simulink model "Phase1_Mark2"  (R2024b)
settings: Solver=ode23tb  StartTime=0.0  StopTime=inf  FixedStep=.001  RelTol=1e-1
model workspace (MAT data in the model file):
  A_mu = 10
  B_reff = 8.386
  CONVERTER_DATA = [0 0.1 0.2 0.3 0.4 0.5 0.6 0.7 0.8 0.81 0.82 0.83 ... (63 elements, 21x3)]
  Cps = 2
  Cz = 7766.25
  DOWN_TABLE = [0 0 0 0 0 0 5 5 7.5 7.5 15 15 ... (30 elements, 6x5)]
  DOWN_TH_BP = [0 5 40 50 90 100]
  D_reff = 0.25826
  EMAP = [-40 215 245 264 264 267 267 267 267 267 -44 117 ... (110 elements, 10x11)]
  F0z = [6086.4 4324.8]
  F_reff = 0.07394
  F_zmax = 10000
  F_zmin = 100
  F_zo = 4000
  Kz = 48000
  MF : object (value not decoded)
  NCyl = 6
  NE_VEC = [800 1200 1600 2000 2400 2800 3200 3600 4000 4400 4800]
  Pstd = 101325
  Rair = 287
  SUS : object (value not decoded)
  TH_VEC = [0; 20; 30; 40; 50; 60; 70; 80; 90; 100]
  TWAITdn = 1.25
  TWAITup = 0.1
  Tin = [1 2 3 4 5 6 7 8 9 10 2 2 ... (20 elements, 10x2)]
  Tstd = 293.15
  UP_TABLE = [7.5 7.5 15 25 40 40 25 25 35 45 70 80 ... (30 elements, 6x5)]
  UP_TH_BP = [0 25 35 50 90 100]
  VEH : object (value not decoded)
  V_o = 16.7
  V_xlow = 1
  Vd = 0.00346
  WH : object (value not decoded)
  a = 1.515
  alpha_max = 1.5
  alpha_min = -1.5
  b = 1.504
  c_zo = 209651
  epsilon = 0.1
  f_air = [0 0 0 0 0 0 0 0 0 0 0 0 ... (256 elements, 16x16)]
  f_co = [0 0 0 0 0 0 0 0 0 0 0 0 ... (256 elements, 16x16)]
  f_co2 = [0 0 0 0 0 0 0 0 0 0 0 0 ... (256 elements, 16x16)]
  f_eff = [352.135682859 352.135682859 320.724378192 303.655312657 295.930136708 291.240087194 291.240271258 291.240312459 291.240275452 291.240198499 291.240100781 291.240018769 ... (256 elements, 16x16)]
  f_fuel = [0 0 0 0 0 0 0 0 0 0 0 0 ... (256 elements, 16x16)]
  f_hc = [0 0 0 0 0 0 0 0 0 0 0 0 ... (256 elements, 16x16)]
  f_nox = [0 0 0 0 0 0 0 0 0 0 0 0 ... (256 elements, 16x16)]
  f_pm = [0 0 0 0 0 0 0 0 0 0 0 0 ... (256 elements, 16x16)]
  f_susp_axl_bp = [1 2]
  f_susp_dz_bp = [-4 -0.14 -0.13 -0.12 -0.11 -0.1 -0.09 -0.08 -0.07 -0.06 -0.05 -0.04 ... (31 elements, 1x31)]
  f_susp_dzdot_bp = [-4 -0.14 -0.13 -0.12 -0.11 -0.1 -0.09 -0.08 -0.07 -0.06 -0.05 -0.04 ... (31 elements, 1x31)]
  f_susp_fmz = [-213379.591456 -28099.591456 -27619.591456 -27139.591456 -26659.591456 -26179.591456 -25699.591456 -25219.591456 -24739.591456 -24259.591456 -23779.591456 -23299.591456 ... (468968 elements, 31x31x61x2x4)]
  f_susp_geom = [-0.832564012244 0.043269987756 0.045538987756 0.047807987756 0.050076987756 0.052345987756 0.054614987756 0.056883987756 0.059152987756 0.061421987756 0.063690987756 0.065959987756 ... (11346 elements, 31x61x2x3)]
  f_susp_strgdelta_bp = [-0.523598775598 -0.506145483078 -0.488692190558 -0.471238898038 -0.453785605519 -0.436332312999 -0.418879020479 -0.401425727959 -0.383972435439 -0.366519142919 -0.349065850399 -0.331612557879 ... (61 elements, 1x61)]
  f_tbrake = [0 76.8593923996 105.140482948 131.533638111 157.926793274 176.658631717 176.65727296 176.656856686 176.656879077 176.657093756 176.657404516 176.65772406 ... (256 elements, 16x16)]
  f_tbrake_n_bpt = [0 649.519052838 912.419621844 1175.32019085 1438.22075986 1701.12132886 1964.02189787 2226.92246687 2489.82303588 2752.72360489 3015.62417389 3278.5247429 ... (16 elements, 1x16)]
  f_tbrake_t_bpt = [0 34.6410161514 61.0341713143 87.4273264773 113.82048164 140.213636803 166.606791966 192.999947129 219.393102292 245.786257455 272.179412618 298.572567781 ... (16 elements, 1x16)]
  f_texh = [766.752464599 766.752464599 786.17542386 801.679939032 884.591982581 910.574397722 910.571871054 910.570774534 910.570601632 910.570821151 910.571247242 910.571639815 ... (256 elements, 16x16)]
  f_twc_eff_co = [0.17 0.25 0.45 0.99 0.99 0.99 0.99]
  f_twc_eff_hc = [0.21 0.375 0.75 0.98 0.98 0.98 0.98]
  f_twc_eff_lam = [0.909090909 0.944055944 0.979020979 1 1.013986014 1.048951049 1.083916084]
  f_twc_eff_nox = [0.98 0.98 0.98 0.97 0.05 0.02 0]
  h = 0.134
  k_z = 50
  kappa_max = 1.5
  kappa_min = -1.5
  lam_Cx = 1
  lam_Cy = 1
  lam_Cz = 1
  lam_Ex = 1
  lam_Ey = 1
  lam_F_zo = 1
  lam_Hx = 1
  lam_Hy = 1
  lam_Kxkappa = 1
  lam_Kyalpha = 1
  lam_Kygamma = 1
  lam_Kzgamma = 1
  lam_Mr = 1
  lam_Mx = 1
  lam_My = 1
  lam_S = 1
  lam_VMx = 1
  lam_Vx = 1
  lam_Vy = 1
  lam_Vykappa = 1
  lam_muV = 0
  lam_mux = 1
  lam_muy = 1
  lam_t = 1
  lam_xalpha = 1
  lam_ykappa = 1
  numWheel = 4
  p_Cx1 = 1.579
  p_Cy1 = 1.3332
  p_Dx1 = 1.0422
  p_Dx2 = -0.08285
  p_Dx3 = 0
  p_Dy1 = 0.8784
  p_Dy2 = -0.06445
  p_Dy3 = 0
  p_Ex1 = 0.11185
  p_Ex2 = 0.3127
  p_Ex3 = 0
  p_Ex4 = 0.001603
  p_Ey1 = -0.8227
  p_Ey2 = -0.6062
  p_Ey3 = 0.09825
  p_Ey4 = -6.546
  p_Ey5 = 0
  p_Fz1 = 0.7098
  p_Hx1 = 0.00021585
  p_Hx2 = 0.0011538
  p_Hy1 = -0.0018043
  p_Hy2 = 0.003518
  p_Kx1 = 21.69
  p_Kx2 = 13.774
  p_Kx3 = -0.4119
  p_Ky1 = -15.314
  p_Ky2 = 1.7044
  p_Ky3 = 0.36986
  p_Ky4 = 1.9896
  p_Ky5 = 0
  p_Ky6 = -0.9004
  p_Ky7 = -0.2328
  p_Vx1 = 1.5973e-05
  p_Vx2 = 0.0001043
  p_Vy1 = -0.006642
  p_Vy2 = 0.03597
  p_Vy3 = -0.1621
  p_Vy4 = -0.4908
  p_pmx1 = 0
  p_px1 = -0.3489
  p_px2 = 0.382
  p_px3 = -0.09634
  p_px4 = 0.06447
  p_py1 = -0.6249
  p_py2 = -0.06535
  p_py3 = -0.1668
  p_py4 = 0.2834
  p_py5 = 0
  path : object (value not decoded)
  pio = 220000
  q_Fcx = 0
  q_Fz2 = 15.4
  q_Fzy = 0
  q_reo = 0.9974
  q_sx1 = -0.007764
  q_sx10 = 0.2824
  q_sx11 = 5.349
  q_sx12 = 0
  q_sx13 = 0
  q_sx14 = 0
  q_sx2 = 1.1915
  q_sx3 = 0.013948
  q_sx4 = 4.912
  q_sx5 = 1.02
  q_sx6 = 22.83
  q_sx7 = 0.7104
  q_sx8 = -0.023393
  q_sx9 = 0.6581
  q_sy1 = 0.00702
  q_sy2 = 0
  q_sy3 = 0.001515
  q_sy4 = 8.514e-05
  q_sy5 = 0
  q_sy6 = 0
  q_sy7 = 0.9008
  q_sy8 = -0.4089
  q_v1 = 0.0007742
  q_v2 = 0.04667
  r_Bx1 = 12.531
  r_Bx2 = 9.532
  r_Bx3 = 0
  r_By1 = 10.615
  r_By2 = 7.705
  r_By3 = 3.433e-06
  r_By4 = 0
  r_Cx1 = 1.019
  r_Cy1 = 1.0585
  r_Ex1 = -0.4487
  r_Ex2 = -0.4726
  r_Ey1 = 0.3132
  r_Ey2 = 7.63e-06
  r_Hx1 = 0.0002374
  r_Hy1 = 0.011646
  r_Hy2 = 7.63e-06
  r_Vy1 = 0.05654
  r_Vy2 = 7.63e-06
  r_Vy3 = 0
  r_Vy4 = 99.9
  r_Vy5 = 2
  r_Vy6 = 15.814
  r_o = 0.3135
  reqTmaxT = [nan 0.285774810084 0.647179872268 nan nan nan nan nan nan nan nan nan ... (168 elements, 21x8)]
  vehSpd = [0 2.77777777778 5.55555555556 8.33333333333 11.1111111111 13.8888888889 16.6666666667 19.4444444444 22.2222222222 25 27.7777777778 30.5555555556 ... (21 elements, 1x21)]
  vehWidth = 2
  w = 1
symbols that are objects in the model workspace (value not decoded): VEH
undefined symbols (not defined in the file or in its folder): Fzz, Fzzdot, InertFrm, pFz, psi, vdyntiremask, x_o, zdotFz, zFz
(part 16 of 24)

== system Phase1_Mark2/Longitudinal Wheels 4DOF/Tires/MF/Combined Slip Wheel 2DOF/Wheel Module/Clutch/Clutch Partitioned Parameters/Clutch/Slipping ==
  Tfmaxk : Inport
  Tout : Inport  Port=2
  f : ActionPort
      settings: CopyFcn=Stateflow.SLINSF.SimulinkMan.removeBlockPreDeleteFcn  PreDeleteFcn=Stateflow.SLINSF.SimulinkMan.unsafePredeleteFcn
  -4 : Gain  Gain=-4  SaturateOnIntegerOverflow=on  OutDataTypeStr=Inherit: Same as input  ParamDataTypeStr=Inherit: Same as input
  Max Dynamic Friction Torque1 : Product  InputSameDT=on  RndMeth=Zero  SaturateOnIntegerOverflow=on  OutDataTypeStr=Inherit: Same as first input
  Output Inertia : Gain  Gain=1./Iyy  SaturateOnIntegerOverflow=on  OutDataTypeStr=Inherit: Same as input  ParamDataTypeStr=Inherit: Same as input
  Output Damping : Gain  Gain=br  SaturateOnIntegerOverflow=on  OutDataTypeStr=Inherit: Same as input  ParamDataTypeStr=Inherit: Same as input
  Output Sum : Sum  Inputs=|+--  InputSameDT=on  SaturateOnIntegerOverflow=on  OutDataTypeStr=Inherit: Same as first input
  Trigonometric Function : Trigonometry  Operator=tanh
  omega wheel : Integrator  InitialCondition=omegao  ContinuousStateAttributes='omegaWheel'
  Omega : Outport  InitialOutput=0  VectorParamsAs1DForOutWhenUnconnected=off
  Omegadot : Outport  Port=2  InitialOutput=0  VectorParamsAs1DForOutWhenUnconnected=off
  ReactionTorque : Outport  Port=3  InitialOutput=0  VectorParamsAs1DForOutWhenUnconnected=off
  Myb : Outport  Port=4  InitialOutput=0  VectorParamsAs1DForOutWhenUnconnected=off
  BrkTrq : Outport  Port=5  InitialOutput=0  VectorParamsAs1DForOutWhenUnconnected=off
  wires:
  omega wheel/1 -> Output Damping/1, -4/1, Omega/1
  Tfmaxk/1 -> Max Dynamic Friction Torque1/1
  Output Inertia/1 -> omega wheel/1, Omegadot/1
  -4/1 -> Trigonometric Function/1
  Trigonometric Function/1 -> Max Dynamic Friction Torque1/2
  Max Dynamic Friction Torque1/1 -> Output Sum/1, BrkTrq/1
  Tout/1 -> Output Sum/2
  Output Sum/1 -> Output Inertia/1, ReactionTorque/1
  Output Damping/1 -> Output Sum/3, Myb/1

== system Phase1_Mark2/Longitudinal Wheels 4DOF/Tires/MF/Combined Slip Wheel 2DOF/Wheel Module/Clutch/Clutch Partitioned Parameters/Clutch/detectLockup ==
  Tout : Inport  OutDataTypeStr=double  PortDimensions=1
  Tfmaxs : Inport  Port=2  OutDataTypeStr=double  PortDimensions=1
  f : TriggerPort  TriggerType=function-call  VariantControl=Variant
      settings: CopyFcn=Stateflow.SLINSF.SimulinkMan.removeBlockPreDeleteFcn  PreDeleteFcn=Stateflow.SLINSF.SimulinkMan.unsafePredeleteFcn
  Constant : Constant  Value=0
  Friction Mode Logic : Subsystem
      mask Display: plot([-3 1 1 3 -1 -1],[-1 -1 1 1 1 -1],-4,-5,4,5)
  yn : Outport  VectorParamsAs1DForOutWhenUnconnected=off
  wires:
  Constant/1 -> Friction Mode Logic/3(locked_wout)
  Friction Mode Logic/1(locked) -> yn/1  "LockedFlag"
  Tout/1 -> Friction Mode Logic/1(Tout)
  Tfmaxs/1 -> Friction Mode Logic/2(Tfmaxs)

== system Phase1_Mark2/Longitudinal Wheels 4DOF/Tires/MF/Combined Slip Wheel 2DOF/Wheel Module/Clutch/Clutch Partitioned Parameters/Clutch/detectSlip ==
  Tout : Inport  OutDataTypeStr=double  PortDimensions=1
  Tfmaxs : Inport  Port=2  OutDataTypeStr=double  PortDimensions=1
  f : TriggerPort  TriggerType=function-call  VariantControl=Variant
      settings: CopyFcn=Stateflow.SLINSF.SimulinkMan.removeBlockPreDeleteFcn  PreDeleteFcn=Stateflow.SLINSF.SimulinkMan.unsafePredeleteFcn
  Break Apart Detection : Subsystem
  yn : Outport  VectorParamsAs1DForOutWhenUnconnected=off
  wires:
  Break Apart Detection/1(unlock) -> yn/1
  Tout/1 -> Break Apart Detection/2(Tf)
  Tfmaxs/1 -> Break Apart Detection/1(Tfmaxs)

== system Phase1_Mark2/Longitudinal Wheels 4DOF/Tires/MF/Combined Slip Wheel 2DOF/Wheel Module/Clutch/Clutch Scalar Parameters/Clutch/Locked ==
  Tout : Inport
  f : ActionPort
      settings: CopyFcn=Stateflow.SLINSF.SimulinkMan.removeBlockPreDeleteFcn  PreDeleteFcn=Stateflow.SLINSF.SimulinkMan.unsafePredeleteFcn
  Constant : Constant  Value=0
  Constant1 : Constant  Value=0
  Constant2 : Constant  Value=0
  Unary Minus : UnaryMinus
  ReactionTorque : Outport  InitialOutput=0  VectorParamsAs1DForOutWhenUnconnected=off
  Omega : Outport  Port=2  InitialOutput=0  VectorParamsAs1DForOutWhenUnconnected=off
  Omegadot : Outport  Port=3  InitialOutput=0  VectorParamsAs1DForOutWhenUnconnected=off
  Myb : Outport  Port=4  InitialOutput=0  VectorParamsAs1DForOutWhenUnconnected=off
  BrkTrq : Outport  Port=5  InitialOutput=0  VectorParamsAs1DForOutWhenUnconnected=off
  wires:
  Constant/1 -> Omega/1
  Constant2/1 -> Myb/1
  Constant1/1 -> Omegadot/1
  Tout/1 -> Unary Minus/1, BrkTrq/1
  Unary Minus/1 -> ReactionTorque/1

== system Phase1_Mark2/Longitudinal Wheels 4DOF/Tires/MF/Combined Slip Wheel 2DOF/Wheel Module/Clutch/Clutch Scalar Parameters/Clutch/Slipping ==
  Tfmaxk : Inport
  Tout : Inport  Port=2
  f : ActionPort
      settings: CopyFcn=Stateflow.SLINSF.SimulinkMan.removeBlockPreDeleteFcn  PreDeleteFcn=Stateflow.SLINSF.SimulinkMan.unsafePredeleteFcn
  -4 : Gain  Gain=-4  SaturateOnIntegerOverflow=on  OutDataTypeStr=Inherit: Same as input  ParamDataTypeStr=Inherit: Same as input
  Max Dynamic Friction Torque1 : Product  InputSameDT=on  RndMeth=Zero  SaturateOnIntegerOverflow=on  OutDataTypeStr=Inherit: Same as first input
  Output Inertia : Gain  Gain=1./Iyy  SaturateOnIntegerOverflow=on  OutDataTypeStr=Inherit: Same as input  ParamDataTypeStr=Inherit: Same as input
  Output Damping : Gain  Gain=br  SaturateOnIntegerOverflow=on  OutDataTypeStr=Inherit: Same as input  ParamDataTypeStr=Inherit: Same as input
  Output Sum : Sum  Inputs=|+--  InputSameDT=on  SaturateOnIntegerOverflow=on  OutDataTypeStr=Inherit: Same as first input
  Trigonometric Function : Trigonometry  Operator=tanh
  omega wheel : Integrator  InitialCondition=omegao  ContinuousStateAttributes='omegaWheel'
  Omega : Outport  InitialOutput=0  VectorParamsAs1DForOutWhenUnconnected=off
  Omegadot : Outport  Port=2  InitialOutput=0  VectorParamsAs1DForOutWhenUnconnected=off
  ReactionTorque : Outport  Port=3  InitialOutput=0  VectorParamsAs1DForOutWhenUnconnected=off
  Myb : Outport  Port=4  InitialOutput=0  VectorParamsAs1DForOutWhenUnconnected=off
  BrkTrq : Outport  Port=5  InitialOutput=0  VectorParamsAs1DForOutWhenUnconnected=off
  wires:
  omega wheel/1 -> Output Damping/1, -4/1, Omega/1
  Tfmaxk/1 -> Max Dynamic Friction Torque1/1
  Output Inertia/1 -> omega wheel/1, Omegadot/1
  -4/1 -> Trigonometric Function/1
  Trigonometric Function/1 -> Max Dynamic Friction Torque1/2
  Max Dynamic Friction Torque1/1 -> Output Sum/1, BrkTrq/1
  Tout/1 -> Output Sum/2
  Output Sum/1 -> Output Inertia/1, ReactionTorque/1
  Output Damping/1 -> Output Sum/3, Myb/1

== system Phase1_Mark2/Longitudinal Wheels 4DOF/Tires/MF/Combined Slip Wheel 2DOF/Wheel Module/Clutch/Clutch Scalar Parameters/Clutch/detectLockup ==
  Tout : Inport  OutDataTypeStr=double  PortDimensions=1
  Tfmaxs : Inport  Port=2  OutDataTypeStr=double  PortDimensions=1
  f : TriggerPort  TriggerType=function-call  VariantControl=Variant
      settings: CopyFcn=Stateflow.SLINSF.SimulinkMan.removeBlockPreDeleteFcn  PreDeleteFcn=Stateflow.SLINSF.SimulinkMan.unsafePredeleteFcn
  Constant : Constant  Value=0
  Friction Mode Logic : Subsystem
      mask Display: plot([-3 1 1 3 -1 -1],[-1 -1 1 1 1 -1],-4,-5,4,5)
  yn : Outport  VectorParamsAs1DForOutWhenUnconnected=off
  wires:
  Constant/1 -> Friction Mode Logic/3(locked_wout)
  Friction Mode Logic/1(locked) -> yn/1  "LockedFlag"
  Tout/1 -> Friction Mode Logic/1(Tout)
  Tfmaxs/1 -> Friction Mode Logic/2(Tfmaxs)

== system Phase1_Mark2/Longitudinal Wheels 4DOF/Tires/MF/Combined Slip Wheel 2DOF/Wheel Module/Clutch/Clutch Scalar Parameters/Clutch/detectSlip ==
  Tout : Inport  OutDataTypeStr=double  PortDimensions=1
  Tfmaxs : Inport  Port=2  OutDataTypeStr=double  PortDimensions=1
  f : TriggerPort  TriggerType=function-call  VariantControl=Variant
      settings: CopyFcn=Stateflow.SLINSF.SimulinkMan.removeBlockPreDeleteFcn  PreDeleteFcn=Stateflow.SLINSF.SimulinkMan.unsafePredeleteFcn
  Break Apart Detection : Subsystem
  yn : Outport  VectorParamsAs1DForOutWhenUnconnected=off
  wires:
  Break Apart Detection/1(unlock) -> yn/1
  Tout/1 -> Break Apart Detection/2(Tf)
  Tfmaxs/1 -> Break Apart Detection/1(Tfmaxs)

== system Phase1_Mark2/Vehicle Body 3DOF External Longitudinal Wheels/Bicycle/Vehicle Body 3DOF Single Track/Signal Routing/Signal Routing/Lateral 3DOF/Hard Point Coordinate Transform Front/Rotation Angles to Direction Cosine Matrix ==
  In1 : Inport  Unit=rad  PortDimensions=3
  Create 3x3 Matrix : Subsystem  mask(Create 3x3 Matrix){aMode=aMode}
      mask help: shared_aeroblks:sharedaeroblkutil:blockCreate3x3MatrixDesc
      mask init:
      | if aerosharedtest(gcb)
      |     aerosharedicon('shared');
      | else
      |     sharedautoicon('shared');
      | end
      mask Help: eval('if license(''test'',''Aerospace_Blockset'')aerosharedhelp(''create_threebythree_matrix'');elseif license(''test'',''Powertrain_Blockset'')sharedautohelp(''create_threebythree_matrix'');end')
      mask Display:
      | port_label('input',1,'A_{11}','texmode','on');
      | port_label('input',2,'A_{12}','texmode','on');
      | port_label('input',3,'A_{13}','texmode','on');
      | port_label('input',4,'A_{21}','texmode','on');
      | port_label('input',5,'A_{22}','texmode','on');
      | port_label('input',6,'A_{23}','texmode','on');
      | port_label('input',7,'A_{31}','texmode','on');
      | port_label('input',8,'A_{32}','texmode','on');
      | port_label('input',9,'A_{33}','texmode','on');
      | port_label('output',1,'A','texmode','on');
  Fcn11 : Fcn  Expr=u(5)*u(4)
  Fcn12 : Fcn  Expr=u(5)*u(1)
  Fcn13 : Fcn  Expr=-u(2)
  Fcn21 : Fcn  Expr=u(3)*u(2)*u(4) - u(6)*u(1)
  Fcn22 : Fcn  Expr=u(3)*u(2)*u(1) + u(6)*u(4)
  Fcn23 : Fcn  Expr=u(3)*u(5)
  Fcn31 : Fcn  Expr=u(6)*u(2)*u(4) + u(3)*u(1)
  Fcn32 : Fcn  Expr=u(6)*u(2)*u(1) - u(3)*u(4)
  Fcn33 : Fcn  Expr=u(6)*u(5)
  Mux : Mux  Inputs=2
  sincos : Trigonometry  Operator=sincos
  Out1 : Outport  Unit=1  PortDimensions=[3,3]  VectorParamsAs1DForOutWhenUnconnected=off
  wires:
  In1/1 -> sincos/1
  Create 3x3 Matrix/1(Matrix) -> Out1/1
  sincos/1 -> Mux/1
  sincos/2 -> Mux/2
  Mux/1 -> Fcn11/1, Fcn12/1, Fcn13/1, Fcn21/1, Fcn32/1, Fcn33/1, Fcn31/1, Fcn23/1, Fcn22/1
  Fcn11/1 -> Create 3x3 Matrix/1(M11)
  Fcn12/1 -> Create 3x3 Matrix/2(M12)
  Fcn13/1 -> Create 3x3 Matrix/3(M13)
  Fcn21/1 -> Create 3x3 Matrix/4(M21)
  Fcn31/1 -> Create 3x3 Matrix/7(M31)
  Fcn22/1 -> Create 3x3 Matrix/5(M22)
  Fcn23/1 -> Create 3x3 Matrix/6(M23)
  Fcn32/1 -> Create 3x3 Matrix/8(M32)
  Fcn33/1 -> Create 3x3 Matrix/9(M33)

== system Phase1_Mark2/Vehicle Body 3DOF External Longitudinal Wheels/Bicycle/Vehicle Body 3DOF Single Track/Signal Routing/Signal Routing/Lateral 3DOF/Hard Point Coordinate Transform Front/transform to Inertial axes ==
  x y z : Inport
  transform coefficients : Inport  Port=2
  Product : Product  Multiplication=Matrix(*)  InputSameDT=on  SaturateOnIntegerOverflow=on  OutDataTypeStr=Inherit: Same as first input
  Reshape1 : Reshape  OutputDimensionality=Column vector (2-D)
  Reshape2 : Reshape
  Ve : Outport  VectorParamsAs1DForOutWhenUnconnected=off
  wires:
  Reshape2/1 -> Ve/1
  Reshape1/1 -> Product/2
  x y z/1 -> Reshape1/1
  transform coefficients/1 -> Product/1
  Product/1 -> Reshape2/1

== system Phase1_Mark2/Vehicle Body 3DOF External Longitudinal Wheels/Bicycle/Vehicle Body 3DOF Single Track/Signal Routing/Signal Routing/Lateral 3DOF/Hard Point Coordinate Transform Front/transform to Inertial axes1 ==
  x y z : Inport
  transform coefficients : Inport  Port=2
  Product : Product  Multiplication=Matrix(*)  InputSameDT=on  SaturateOnIntegerOverflow=on  OutDataTypeStr=Inherit: Same as first input
  Reshape1 : Reshape  OutputDimensionality=Column vector (2-D)
  Reshape2 : Reshape
  Ve : Outport  VectorParamsAs1DForOutWhenUnconnected=off
  wires:
  Reshape2/1 -> Ve/1
  Reshape1/1 -> Product/2
  x y z/1 -> Reshape1/1
  transform coefficients/1 -> Product/1
  Product/1 -> Reshape2/1

== system Phase1_Mark2/Vehicle Body 3DOF External Longitudinal Wheels/Bicycle/Vehicle Body 3DOF Single Track/Signal Routing/Signal Routing/Lateral 3DOF/Hard Point Coordinate Transform Front/wxR ==
  A : Inport
  B : Inport  Port=2
  "A " : InportShadow
  "B " : InportShadow  Port=2
  Subsystem : Subsystem
  Subsystem1 : Subsystem
  Sum : Sum  Inputs=+|-  InputSameDT=on  SaturateOnIntegerOverflow=on  OutDataTypeStr=Inherit: Same as first input
  C : Outport  VectorParamsAs1DForOutWhenUnconnected=off
  wires:
  "B "/1 -> Subsystem1/2(B)
  "A "/1 -> Subsystem1/1(A)
  Sum/1 -> C/1
  B/1 -> Subsystem/2(B)
  A/1 -> Subsystem/1(A)
  Subsystem/1(Out1) -> Sum/1
  Subsystem1/1(Out1) -> Sum/2

== system Phase1_Mark2/Vehicle Body 3DOF External Longitudinal Wheels/Bicycle/Vehicle Body 3DOF Single Track/Signal Routing/Signal Routing/Lateral 3DOF/Hard Point Coordinate Transform Geometric/Hard Point Coordinate Transform External Displacement Beta ==
  InertFrmCg : Inport
  BdyFrmCg : Inport  Port=2
  R : Inport  Port=3  Unit=m
  Add : Sum
  Add1 : Sum
  Add4 : Sum
  Body Slip : Subsystem
  Bus Creator{1..3,6,10} (5 alike) : BusCreator  Inputs=3
  Bus Creator4 : BusCreator  Inputs=1
  Bus Creator7 : BusCreator  Inputs=2
  Bus Selector1 : BusSelector  OutputSignals=Vel.xdot,Vel.ydot,Vel.zdot  OutputAsBus=on
  Bus Selector4 : BusSelector  OutputSignals=Disp.X,Disp.Y,Disp.Z  OutputAsBus=on
  Bus Selector5 : BusSelector  OutputSignals=AngVel.p,AngVel.q,AngVel.r  OutputAsBus=on
  Bus Selector6 : BusSelector  OutputSignals=Vel.Xdot,Vel.Ydot,Vel.Zdot  OutputAsBus=on
  Bus Selector8 : BusSelector  OutputSignals=Ang.phi,Ang.theta,Ang.psi  OutputAsBus=on
  Bus to Vector{,1..4} (5 alike) : BusToVector
  Demux{1..4} (4 alike) : Demux  Outputs=3
  Rotation Angles to Direction Cosine Matrix : Subsystem  mask(Ang2DCM){rotationOrder=ZYX, aMode=aMode}
      mask prompts: rotationOrder "shared_aeroblks:sharedaeroblktransform:blockAng2DCMParamRotationOrder"
      mask help: shared_aeroblks:sharedaeroblktransform:blockAng2DCMDesc
      mask init:
      | if aerosharedtest(gcb)
      |     ports=aerosharedicon('sharedang2dcm');
      | else
      |     ports=sharedautoicon('sharedang2dcm');
      | end
      settings: AttributesFormatString=Rotation Order: %<rotationOrder>
      mask Help: eval('if license(''test'',''Aerospace_Blockset'')aerosharedhelp(''rotation_angles_to_direction_cosine_matrix'');elseif license(''test'',''Powertrain_Blockset'')sharedautohelp(''rotation_angles_to_direction_cosine_matrix'');end')
      mask TypeOptions rotationOrder: shared_aeroblks:sharedaeroblktransform:blockParamComboZYX | shared_aeroblks:sharedaeroblktransform:blockParamComboZYZ | shared_aeroblks:sharedaeroblktransform:blockParamComboZXY | shared_aeroblks:sharedaeroblktransform:blockParamComboZXZ | shared_aeroblks:sharedaeroblktransform:blockParamComboYXZ | shared_aeroblks:sharedaeroblktransform:blockParamComboYXY | shared_aeroblks:sharedaeroblktransform:blockParamComboYZX | shared_aeroblks:sharedaeroblktransform:blockParamComboYZY | shared_aeroblks:sharedaeroblktransform:blockParamComboXYZ | shared_aeroblks:sharedaeroblktransform:blockParamComboXYX | shared_aeroblks:sharedaeroblktransform:blockParamComboXZY | shared_aeroblks:sharedaeroblktransform:blockParamComboXZX
      mask DialogControl rotationOrder Prompt: Rotation order:
      mask Display:
      | port_label('input',1,'[R_1,R_2,R_3]','texmode','on')
      | port_label('output',1,'DCM_{be}','texmode','on')
  Selector1 : Selector  InputPortWidth=3  IndexOptions=Index vector (dialog)  Indices=[3 2 1]  OutputSizes=1
  Signal Specification : SignalSpecification  Unit=m
  Signal Specification1 : SignalSpecification  Unit=m
  Signal Specification2 : SignalSpecification  Unit=m/s
  Signal Specification3 : SignalSpecification  Unit=m/s
  Transpose1 : Math  Operator=transpose  SignedPower=on
  transform to Inertial axes : Subsystem  mask(Vector Transformation){}
      mask Display: disp('L_EB')
  transform to Inertial axes1 : Subsystem  mask(Vector Transformation){}
      mask Display: disp('L_EB')
  wxR : Subsystem  mask(CrossProduct){aMode=aMode}
      mask help: shared_aeroblks:sharedaeroblkutil:blockCrossProductDesc
      mask init:
      | if aerosharedtest(gcb)
      |     aerosharedicon('shared');
      | else
      |     sharedautoicon('shared');
      | end
      mask Help: eval('if license(''test'',''Aerospace_Blockset'')aerosharedhelp(''threebythree_cross_product'');elseif license(''test'',''Powertrain_Blockset'')sharedautohelp(''threebythree_cross_product'');end')
      mask Display:
      | text(.5,.5,'Cross\nProduct\nC = AxB', ...
      | 	'HorizontalAlignment','Center',...
      | 	'VerticalAlignment','middle')
  Inertial : Outport  VectorParamsAs1DForOutWhenUnconnected=off
  Body : Outport  Port=2  VectorParamsAs1DForOutWhenUnconnected=off
  wires:
  Signal Specification3/1 -> Demux4/1
  Signal Specification2/1 -> Demux2/1
  Signal Specification1/1 -> Demux3/1
  Signal Specification/1 -> Demux1/1
  R/1 -> Signal Specification1/1, transform to Inertial axes1/1(x y z), wxR/2(B)
  Bus to Vector3/1 -> Add1/2
  Add1/1 -> Signal Specification3/1, Body Slip/1(x)
  Bus Selector1/1 -> Bus to Vector3/1
  Bus Creator3/1 -> Body/1
  Demux4/2 -> Bus Creator2/2  "ydot"
  Demux3/2 -> Bus Creator1/2  "y"
  Demux3/3 -> Bus Creator1/3  "z"
  Demux3/1 -> Bus Creator1/1  "x"
  Demux4/3 -> Bus Creator2/3  "zdot"
  Demux4/1 -> Bus Creator2/1  "xdot"
  Bus Creator2/1 -> Bus Creator3/2  "Vel"
  Bus Creator1/1 -> Bus Creator3/1  "Disp"
  Bus Creator7/1 -> Inertial/1
  Demux2/2 -> Bus Creator6/2  "Ydot"
  Demux1/2 -> Bus Creator10/2  "Y"
  Demux1/3 -> Bus Creator10/3  "Z"
  Demux1/1 -> Bus Creator10/1  "X"
  Demux2/3 -> Bus Creator6/3  "Zdot"
  Demux2/1 -> Bus Creator6/1  "Xdot"
  Bus Creator6/1 -> Bus Creator7/2  "Vel"
  Bus Creator10/1 -> Bus Creator7/1  "Disp"
  transform to Inertial axes1/1(Ve) -> Add/2
  Bus to Vector4/1 -> Selector1/1
  Bus Selector8/1 -> Bus to Vector4/1
  Rotation Angles to Direction Cosine Matrix/1(Out1) -> Transpose1/1
  Selector1/1 -> Rotation Angles to Direction Cosine Matrix/1(In1)
  Transpose1/1 -> transform to Inertial axes/2(transform coefficients), transform to Inertial axes1/2(transform coefficients)
  wxR/1(C) -> Add1/1, transform to Inertial axes/1(x y z)
  Bus to Vector1/1 -> Add4/1  "Vo"
  transform to Inertial axes/1(Ve) -> Add4/2
  Bus to Vector/1 -> wxR/1(A)
  Bus Selector5/1 -> Bus to Vector/1
  Bus Selector6/1 -> Bus to Vector1/1
  Add4/1 -> Signal Specification2/1  "V_wb"
  Add/1 -> Signal Specification/1
  Bus Selector4/1 -> Bus to Vector2/1
  Bus to Vector2/1 -> Add/1
  InertFrmCg/1 -> Bus Selector4/1, Bus Selector6/1, Bus Selector8/1
  BdyFrmCg/1 -> Bus Selector5/1, Bus Selector1/1
  Body Slip/1(Beta) -> Bus Creator4/1  "Beta"
  Bus Creator4/1 -> Bus Creator3/3  "Ang"

== system Phase1_Mark2/Vehicle Body 3DOF External Longitudinal Wheels/Bicycle/Vehicle Body 3DOF Single Track/Signal Routing/Signal Routing/Lateral 3DOF/Hard Point Coordinate Transform Rear/Rotation Angles to Direction Cosine Matrix ==
  In1 : Inport  Unit=rad  PortDimensions=3
  Create 3x3 Matrix : Subsystem  mask(Create 3x3 Matrix){aMode=aMode}
      mask help: shared_aeroblks:sharedaeroblkutil:blockCreate3x3MatrixDesc
      mask init:
      | if aerosharedtest(gcb)
      |     aerosharedicon('shared');
      | else
      |     sharedautoicon('shared');
      | end
      mask Help: eval('if license(''test'',''Aerospace_Blockset'')aerosharedhelp(''create_threebythree_matrix'');elseif license(''test'',''Powertrain_Blockset'')sharedautohelp(''create_threebythree_matrix'');end')
      mask Display:
      | port_label('input',1,'A_{11}','texmode','on');
      | port_label('input',2,'A_{12}','texmode','on');
      | port_label('input',3,'A_{13}','texmode','on');
      | port_label('input',4,'A_{21}','texmode','on');
      | port_label('input',5,'A_{22}','texmode','on');
      | port_label('input',6,'A_{23}','texmode','on');
      | port_label('input',7,'A_{31}','texmode','on');
      | port_label('input',8,'A_{32}','texmode','on');
      | port_label('input',9,'A_{33}','texmode','on');
      | port_label('output',1,'A','texmode','on');
  Fcn11 : Fcn  Expr=u(5)*u(4)
  Fcn12 : Fcn  Expr=u(5)*u(1)
  Fcn13 : Fcn  Expr=-u(2)
  Fcn21 : Fcn  Expr=u(3)*u(2)*u(4) - u(6)*u(1)
  Fcn22 : Fcn  Expr=u(3)*u(2)*u(1) + u(6)*u(4)
  Fcn23 : Fcn  Expr=u(3)*u(5)
  Fcn31 : Fcn  Expr=u(6)*u(2)*u(4) + u(3)*u(1)
  Fcn32 : Fcn  Expr=u(6)*u(2)*u(1) - u(3)*u(4)
  Fcn33 : Fcn  Expr=u(6)*u(5)
  Mux : Mux  Inputs=2
  sincos : Trigonometry  Operator=sincos
  Out1 : Outport  Unit=1  PortDimensions=[3,3]  VectorParamsAs1DForOutWhenUnconnected=off
  wires:
  In1/1 -> sincos/1
  Create 3x3 Matrix/1(Matrix) -> Out1/1
  sincos/1 -> Mux/1
  sincos/2 -> Mux/2
  Mux/1 -> Fcn11/1, Fcn12/1, Fcn13/1, Fcn21/1, Fcn32/1, Fcn33/1, Fcn31/1, Fcn23/1, Fcn22/1
  Fcn11/1 -> Create 3x3 Matrix/1(M11)
  Fcn12/1 -> Create 3x3 Matrix/2(M12)
  Fcn13/1 -> Create 3x3 Matrix/3(M13)
  Fcn21/1 -> Create 3x3 Matrix/4(M21)
  Fcn31/1 -> Create 3x3 Matrix/7(M31)
  Fcn22/1 -> Create 3x3 Matrix/5(M22)
  Fcn23/1 -> Create 3x3 Matrix/6(M23)
  Fcn32/1 -> Create 3x3 Matrix/8(M32)
  Fcn33/1 -> Create 3x3 Matrix/9(M33)

== system Phase1_Mark2/Vehicle Body 3DOF External Longitudinal Wheels/Bicycle/Vehicle Body 3DOF Single Track/Signal Routing/Signal Routing/Lateral 3DOF/Hard Point Coordinate Transform Rear/transform to Inertial axes ==
  x y z : Inport
  transform coefficients : Inport  Port=2
  Product : Product  Multiplication=Matrix(*)  InputSameDT=on  SaturateOnIntegerOverflow=on  OutDataTypeStr=Inherit: Same as first input
  Reshape1 : Reshape  OutputDimensionality=Column vector (2-D)
  Reshape2 : Reshape
  Ve : Outport  VectorParamsAs1DForOutWhenUnconnected=off
  wires:
  Reshape2/1 -> Ve/1
  Reshape1/1 -> Product/2
  x y z/1 -> Reshape1/1
  transform coefficients/1 -> Product/1
  Product/1 -> Reshape2/1

== system Phase1_Mark2/Vehicle Body 3DOF External Longitudinal Wheels/Bicycle/Vehicle Body 3DOF Single Track/Signal Routing/Signal Routing/Lateral 3DOF/Hard Point Coordinate Transform Rear/transform to Inertial axes1 ==
  x y z : Inport
  transform coefficients : Inport  Port=2
  Product : Product  Multiplication=Matrix(*)  InputSameDT=on  SaturateOnIntegerOverflow=on  OutDataTypeStr=Inherit: Same as first input
  Reshape1 : Reshape  OutputDimensionality=Column vector (2-D)
  Reshape2 : Reshape
  Ve : Outport  VectorParamsAs1DForOutWhenUnconnected=off
  wires:
  Reshape2/1 -> Ve/1
  Reshape1/1 -> Product/2
  x y z/1 -> Reshape1/1
  transform coefficients/1 -> Product/1
  Product/1 -> Reshape2/1

== system Phase1_Mark2/Vehicle Body 3DOF External Longitudinal Wheels/Bicycle/Vehicle Body 3DOF Single Track/Signal Routing/Signal Routing/Lateral 3DOF/Hard Point Coordinate Transform Rear/wxR ==
  A : Inport
  B : Inport  Port=2
  "A " : InportShadow
  "B " : InportShadow  Port=2
  Subsystem : Subsystem
  Subsystem1 : Subsystem
  Sum : Sum  Inputs=+|-  InputSameDT=on  SaturateOnIntegerOverflow=on  OutDataTypeStr=Inherit: Same as first input
  C : Outport  VectorParamsAs1DForOutWhenUnconnected=off
  wires:
  "B "/1 -> Subsystem1/2(B)
  "A "/1 -> Subsystem1/1(A)
  Sum/1 -> C/1
  B/1 -> Subsystem/2(B)
  A/1 -> Subsystem/1(A)
  Subsystem/1(Out1) -> Sum/1
  Subsystem1/1(Out1) -> Sum/2

== system Phase1_Mark2/Vehicle Body 3DOF External Longitudinal Wheels/Bicycle/Vehicle Body 3DOF Single Track/Signal Routing/Signal Routing/Lateral 3DOF/Hitch Coordinate Transform/Hard Point Coordinate Transform External Displacement ==
  InertFrmCg : Inport
  BdyFrmCg : Inport  Port=2
  R : Inport  Port=3  Unit=m
  Add : Sum
  Add1 : Sum
  Add4 : Sum
  Bus Creator{1..2,6,10} (4 alike) : BusCreator  Inputs=3
  Bus Creator3 : BusCreator  Inputs=2
  Bus Creator7 : BusCreator  Inputs=2
  Bus Selector1 : BusSelector  OutputSignals=Vel.xdot,Vel.ydot,Vel.zdot  OutputAsBus=on
  Bus Selector4 : BusSelector  OutputSignals=Disp.X,Disp.Y,Disp.Z  OutputAsBus=on
  Bus Selector5 : BusSelector  OutputSignals=AngVel.p,AngVel.q,AngVel.r  OutputAsBus=on
  Bus Selector6 : BusSelector  OutputSignals=Vel.Xdot,Vel.Ydot,Vel.Zdot  OutputAsBus=on
  Bus Selector8 : BusSelector  OutputSignals=Ang.phi,Ang.theta,Ang.psi  OutputAsBus=on
  Bus to Vector{,1..4} (5 alike) : BusToVector
  Demux{1..4} (4 alike) : Demux  Outputs=3
  Rotation Angles to Direction Cosine Matrix : Subsystem  mask(Ang2DCM){rotationOrder=ZYX, aMode=aMode}
      mask prompts: rotationOrder "shared_aeroblks:sharedaeroblktransform:blockAng2DCMParamRotationOrder"
      mask help: shared_aeroblks:sharedaeroblktransform:blockAng2DCMDesc
      mask init:
      | if aerosharedtest(gcb)
      |     ports=aerosharedicon('sharedang2dcm');
      | else
      |     ports=sharedautoicon('sharedang2dcm');
      | end
      settings: AttributesFormatString=Rotation Order: %<rotationOrder>
      mask Help: eval('if license(''test'',''Aerospace_Blockset'')aerosharedhelp(''rotation_angles_to_direction_cosine_matrix'');elseif license(''test'',''Powertrain_Blockset'')sharedautohelp(''rotation_angles_to_direction_cosine_matrix'');end')
      mask TypeOptions rotationOrder: shared_aeroblks:sharedaeroblktransform:blockParamComboZYX | shared_aeroblks:sharedaeroblktransform:blockParamComboZYZ | shared_aeroblks:sharedaeroblktransform:blockParamComboZXY | shared_aeroblks:sharedaeroblktransform:blockParamComboZXZ | shared_aeroblks:sharedaeroblktransform:blockParamComboYXZ | shared_aeroblks:sharedaeroblktransform:blockParamComboYXY | shared_aeroblks:sharedaeroblktransform:blockParamComboYZX | shared_aeroblks:sharedaeroblktransform:blockParamComboYZY | shared_aeroblks:sharedaeroblktransform:blockParamComboXYZ | shared_aeroblks:sharedaeroblktransform:blockParamComboXYX | shared_aeroblks:sharedaeroblktransform:blockParamComboXZY | shared_aeroblks:sharedaeroblktransform:blockParamComboXZX
      mask DialogControl rotationOrder Prompt: Rotation order:
      mask Display:
      | port_label('input',1,'[R_1,R_2,R_3]','texmode','on')
      | port_label('output',1,'DCM_{be}','texmode','on')
  Selector1 : Selector  InputPortWidth=3  IndexOptions=Index vector (dialog)  Indices=[3 2 1]  OutputSizes=1
  Signal Specification : SignalSpecification  Unit=m
  Signal Specification1 : SignalSpecification  Unit=m
  Signal Specification2 : SignalSpecification  Unit=m/s
  Signal Specification3 : SignalSpecification  Unit=m/s
  Transpose1 : Math  Operator=transpose  SignedPower=on
  transform to Inertial axes : Subsystem  mask(Vector Transformation){}
      mask Display: disp('L_EB')
  transform to Inertial axes1 : Subsystem  mask(Vector Transformation){}
      mask Display: disp('L_EB')
  wxR : Subsystem  mask(CrossProduct){aMode=aMode}
      mask help: shared_aeroblks:sharedaeroblkutil:blockCrossProductDesc
      mask init:
      | if aerosharedtest(gcb)
      |     aerosharedicon('shared');
      | else
      |     sharedautoicon('shared');
      | end
      mask Help: eval('if license(''test'',''Aerospace_Blockset'')aerosharedhelp(''threebythree_cross_product'');elseif license(''test'',''Powertrain_Blockset'')sharedautohelp(''threebythree_cross_product'');end')
      mask Display:
      | text(.5,.5,'Cross\nProduct\nC = AxB', ...
      | 	'HorizontalAlignment','Center',...
      | 	'VerticalAlignment','middle')
  Inertial : Outport  VectorParamsAs1DForOutWhenUnconnected=off
  Body : Outport  Port=2  VectorParamsAs1DForOutWhenUnconnected=off
  wires:
  BdyFrmCg/1 -> Bus Selector1/1, Bus Selector5/1
  InertFrmCg/1 -> Bus Selector8/1, Bus Selector6/1, Bus Selector4/1
  Bus to Vector2/1 -> Add/1
  Bus Selector4/1 -> Bus to Vector2/1
  Add/1 -> Signal Specification/1
  Add4/1 -> Signal Specification2/1  "V_wb"
  Bus Selector6/1 -> Bus to Vector1/1
  Bus Selector5/1 -> Bus to Vector/1
  Bus to Vector/1 -> wxR/1(A)
  transform to Inertial axes/1(Ve) -> Add4/2
  Bus to Vector1/1 -> Add4/1  "Vo"
  wxR/1(C) -> transform to Inertial axes/1(x y z), Add1/1
  Transpose1/1 -> transform to Inertial axes1/2(transform coefficients), transform to Inertial axes/2(transform coefficients)
  Selector1/1 -> Rotation Angles to Direction Cosine Matrix/1(In1)
  Rotation Angles to Direction Cosine Matrix/1(Out1) -> Transpose1/1
  Bus Selector8/1 -> Bus to Vector4/1
  Bus to Vector4/1 -> Selector1/1
  transform to Inertial axes1/1(Ve) -> Add/2
  Bus Creator10/1 -> Bus Creator7/1  "Disp"
  Bus Creator6/1 -> Bus Creator7/2  "Vel"
  Demux2/1 -> Bus Creator6/1  "Xdot"
  Demux2/3 -> Bus Creator6/3  "Zdot"
  Demux1/1 -> Bus Creator10/1  "X"
  Demux1/3 -> Bus Creator10/3  "Z"
  Demux1/2 -> Bus Creator10/2  "Y"
  Demux2/2 -> Bus Creator6/2  "Ydot"
  Bus Creator7/1 -> Inertial/1
  Bus Creator1/1 -> Bus Creator3/1  "Disp"
  Bus Creator2/1 -> Bus Creator3/2  "Vel"
  Demux4/1 -> Bus Creator2/1  "xdot"
  Demux4/3 -> Bus Creator2/3  "zdot"
  Demux3/1 -> Bus Creator1/1  "x"
  Demux3/3 -> Bus Creator1/3  "z"
  Demux3/2 -> Bus Creator1/2  "y"
  Demux4/2 -> Bus Creator2/2  "ydot"
  Bus Creator3/1 -> Body/1
  Bus Selector1/1 -> Bus to Vector3/1
  Add1/1 -> Signal Specification3/1
  Bus to Vector3/1 -> Add1/2
  R/1 -> wxR/2(B), transform to Inertial axes1/1(x y z), Signal Specification1/1
  Signal Specification/1 -> Demux1/1
  Signal Specification1/1 -> Demux3/1
  Signal Specification2/1 -> Demux2/1
  Signal Specification3/1 -> Demux4/1

== system Phase1_Mark2/Vehicle Body 3DOF External Longitudinal Wheels/Bicycle/Vehicle Body 3DOF Single Track/Signal Routing/Signal Routing/Power/Power Accounting Bus Creator/PwrNotTrnsfrd Input ==
  PwrIn : Inport
  PwrOut : Outport  VectorParamsAs1DForOutWhenUnconnected=off
  wires:
  PwrIn/1 -> PwrOut/1

== system Phase1_Mark2/Vehicle Body 3DOF External Longitudinal Wheels/Bicycle/Vehicle Body 3DOF Single Track/Signal Routing/Signal Routing/Power/Power Accounting Bus Creator/PwrStored Input ==
  PwrIn : Inport
  PwrOut : Outport  VectorParamsAs1DForOutWhenUnconnected=off
  wires:
  PwrIn/1 -> PwrOut/1

== system Phase1_Mark2/Vehicle Body 3DOF External Longitudinal Wheels/Bicycle/Vehicle Body 3DOF Single Track/Signal Routing/Signal Routing/Power/Power Accounting Bus Creator/PwrTrnsfrd Input ==
  PwrIn : Inport
  PwrOut : Outport  VectorParamsAs1DForOutWhenUnconnected=off
  wires:
  PwrIn/1 -> PwrOut/1

== system Phase1_Mark2/Vehicle Body 3DOF External Longitudinal Wheels/Bicycle/Vehicle Body 3DOF Single Track/Signal Routing/Signal Routing/Power/xdot mode/FxIn ==
  PFExt : Inport
  PMExt : Inport  Port=2
  PFh : Inport  Port=3
  PMh : Inport  Port=4
  PFDrag : Inport  Port=5
  PFwF : Inport  Port=6
  PFwR : Inport  Port=7
  BodyFrm : Inport  Port=8
  Bus Selector2 : BusSelector  OutputSignals=Cg.Acc.ax
  Selector1 : Selector  InputPortWidth=3  IndexOptions=Index vector (dialog)  Indices=[1 2]  OutputSizes=1
  Selector2 : Selector  InputPortWidth=3  IndexOptions=Index vector (dialog)  Indices=[3]  OutputSizes=1
  Selector3 : Selector  InputPortWidth=3  IndexOptions=Index vector (dialog)  Indices=[3]  OutputSizes=1
  Selector4 : Selector  InputPortWidth=3  IndexOptions=Index vector (dialog)  Indices=[1 2]  OutputSizes=1
  Sum : Sum  Inputs=|++
  Sum1 : Sum  Inputs=|++
  Terminator : Terminator
  Terminator2 : Terminator
  Terminator3 : Terminator
  PF : Outport  VectorParamsAs1DForOutWhenUnconnected=off
  PM : Outport  Port=2  VectorParamsAs1DForOutWhenUnconnected=off
  ax : Outport  Port=3  VectorParamsAs1DForOutWhenUnconnected=off
  wires:
  Sum1/1 -> PF/1
  Selector4/1 -> Sum1/2
  PFh/1 -> Selector4/1
  Selector2/1 -> Sum/2
  Sum/1 -> PM/1
  PMh/1 -> Selector2/1
  PFExt/1 -> Selector1/1
  PMExt/1 -> Selector3/1
  PFDrag/1 -> Terminator/1
  Selector3/1 -> Sum/1
  Selector1/1 -> Sum1/1
  PFwR/1 -> Terminator3/1
  PFwF/1 -> Terminator2/1
  BodyFrm/1 -> Bus Selector2/1
  Bus Selector2/1 -> ax/1  "<ax>"

== system Phase1_Mark2/Vehicle Body 3DOF External Longitudinal Wheels/Bicycle/Vehicle Body 3DOF Single Track/Signal Routing/Signal Routing/Power/xdot mode/xdotin ==
  PFExt : Inport
  PMExt : Inport  Port=2
  PFh : Inport  Port=3
  PMh : Inport  Port=4
  PFDrag : Inport  Port=5
  PFwF : Inport  Port=6
  PFwR : Inport  Port=7
  BodyFrm : Inport  Port=8
  Add : Sum  Inputs=+++++
  Ground{,1..5} (6 alike) : Ground
  Mux{,1..4} (5 alike) : Mux  Inputs=2
  Selector1 : Selector  InputPortWidth=3  IndexOptions=Index vector (dialog)  Indices=[1]  OutputSizes=1
  Selector2 : Selector  InputPortWidth=3  IndexOptions=Index vector (dialog)  Indices=[2]  OutputSizes=1
  Selector3 : Selector  InputPortWidth=3  IndexOptions=Index vector (dialog)  Indices=[3]  OutputSizes=1
  Selector4 : Selector  InputPortWidth=3  IndexOptions=Index vector (dialog)  Indices=[1]  OutputSizes=1
  Selector5 : Selector  InputPortWidth=3  IndexOptions=Index vector (dialog)  Indices=[1]  OutputSizes=1
  Selector6 : Selector  InputPortWidth=3  IndexOptions=Index vector (dialog)  Indices=[2]  OutputSizes=1
  Selector7 : Selector  InputPortWidth=3  IndexOptions=Index vector (dialog)  Indices=[3]  OutputSizes=1
  Signal Specification : SignalSpecification  Unit=gn
  Sum : Sum  Inputs=|++
  Terminator : Terminator
  Unary Minus1 : UnaryMinus
  Unary Minus2 : UnaryMinus
  Unary Minus3 : UnaryMinus
  PF : Outport  VectorParamsAs1DForOutWhenUnconnected=off
  PM : Outport  Port=2  VectorParamsAs1DForOutWhenUnconnected=off
  ax : Outport  Port=3  VectorParamsAs1DForOutWhenUnconnected=off
  wires:
  Selector7/1 -> Sum/2
  Sum/1 -> PM/1
  PMh/1 -> Selector7/1
  PFh/1 -> Selector6/1
  Mux4/1 -> Add/4
  Ground5/1 -> Mux4/1
  Selector6/1 -> Mux4/2
  Add/1 -> PF/1
  PMExt/1 -> Selector3/1
  PFExt/1 -> Selector2/1
  PFDrag/1 -> Selector1/1
  Selector1/1 -> Unary Minus3/1
  Selector2/1 -> Mux/2
  Ground/1 -> Mux/1
  Mux/1 -> Add/3
  PFwF/1 -> Selector4/1
  PFwR/1 -> Selector5/1
  Ground1/1 -> Mux2/2
  Selector4/1 -> Unary Minus1/1
  Ground2/1 -> Mux1/2
  Selector5/1 -> Unary Minus2/1
  Mux2/1 -> Add/2
  Mux1/1 -> Add/1
  Unary Minus1/1 -> Mux1/1
  Unary Minus2/1 -> Mux2/1
  Ground3/1 -> Mux3/2
  Mux3/1 -> Add/5
  Selector3/1 -> Sum/1
  Unary Minus3/1 -> Mux3/1
  BodyFrm/1 -> Terminator/1
  Ground4/1 -> Signal Specification/1
  Signal Specification/1 -> ax/1

== system Phase1_Mark2/Vehicle Body 3DOF External Longitudinal Wheels/Bicycle/Vehicle Body 3DOF Single Track/Signal Routing/Signal Routing/state2bus/Angle Wrap/None ==
  u : Inport
  y : Outport  VectorParamsAs1DForOutWhenUnconnected=off
  wires:
  u/1 -> y/1

== system Phase1_Mark2/Vehicle Body 3DOF External Longitudinal Wheels/Bicycle/Vehicle Body 3DOF Single Track/Signal Routing/Signal Routing/state2bus/Angle Wrap/Wrap ==
  u : Inport
  Abs2 : Abs  SaturateOnIntegerOverflow=off
  Add1 : Sum  Inputs=-+
  Constant2 : Constant  Value=pi
  Constant3 : Constant  Value=2
  Divide1 : Product  Inputs=*/
  Floor1 : Rounding
  Gain : Gain  Gain=pi
  Math Function1 : Math  Operator=mod  SignedPower=on
  Math Function3 : Math  Operator=mod  SignedPower=on
  Product1 : Product
  Sign2 : Signum
  Switch : Switch  Criteria=u2 > Threshold  SaturateOnIntegerOverflow=off  InputSameDT=off
  y : Outport  VectorParamsAs1DForOutWhenUnconnected=off
  wires:
  Gain/1 -> Add1/1
  Math Function3/1 -> Switch/2
  Constant3/1 -> Math Function3/2
  Sign2/1 -> Gain/1, Product1/1
  Math Function1/1 -> Product1/2
  Floor1/1 -> Math Function3/1  "N"
  Constant2/1 -> Divide1/2, Math Function1/2
  Divide1/1 -> Floor1/1
  Abs2/1 -> Divide1/1, Math Function1/1
  u/1 -> Abs2/1, Sign2/1
  Product1/1 -> Add1/2, Switch/3
  Add1/1 -> Switch/1
  Switch/1 -> y/1

== system Phase1_Mark2/Vehicle Body 3DOF External Longitudinal Wheels/Bicycle/Vehicle Body 3DOF Single Track/Signal Routing/Signal Routing/state2bus/Body Slip/div0protect - abs poly ==
  u : Inport
  Abs : Abs  ZeroCross=off  SaturateOnIntegerOverflow=off
  Compare To Constant : Subsystem  mask(Compare To Constant){relop=>=, const=-thresh, OutDataTypeStr=boolean, ZeroCross=off}
      mask prompts: relop "Simulink:masks:Operator_MP"; const "Simulink:masks:ConstantValue_MP"; OutDataTypeStr "Simulink:masks:OutputDataType_MP"; ZeroCross "Simulink:masks:EnableZerocrossingDetection_MP"
      mask help: Simulink:masks:CompareToConstant_MD
      mask init:
      | blkName = gcb;
      | 
      | if strcmp(get_param(gcbh,'OutDataTypeStr'),'boolean')
      | 	setValue = 'boolean';
      | else
      | 	setValue = 'fixdt(0, 8, 0)';
      | end
      | 
      | set_param([blkName,'/Compare'],'relop',relop, ...
      | 	'OutDataTypeStr', setValue, 'ZeroCross', ZeroCross);
      | 
      | str = [relop,' C']; %default
      | 
      | const_str = get_param(blkName, 'const');
      | const_val = str2num(const_str);
      | 
      | if isempty(const_val) %#ok<ST2NM>
      |     %Expression/Variable
      |     str = [relop, ' ', strtrim(const_str)];
      | else
      |     if length(const_val) == 1 
      |         if Simulink.data.isSupportedEnumClass(class(const_val))
      |             % Special Handling for Enumerations
      |             if Simulink.data.getEnumTypeInfo(class(const_val), 'AddClassNameToEnumNames')
      |                 str = [relop, ' ', strtrim(const_str)];
      |             else
      |                 str = [relop, ' ', char(const_val)];
      |             end
      |         elseif(isfloat(const_val) || isinteger(const_val) || islogical(const_val)) 
      |                 str = [relop, ' ', num2str(const_val)];
      |         end
      |     end
      | end
      mask TypeOptions relop: == | ~= | < | <= | >= | >
      mask TypeOptions OutDataTypeStr: Simulink:masks:uint8 | Simulink:masks:boolean
      mask Callback ZeroCross: sl('zeroCrossEnable', gcbh);
      mask Display: disp(str)
  Compare To Constant1 : Subsystem  mask(Compare To Constant){relop=<=, const=thresh, OutDataTypeStr=boolean, ZeroCross=off}
      mask prompts: relop "Simulink:masks:Operator_MP"; const "Simulink:masks:ConstantValue_MP"; OutDataTypeStr "Simulink:masks:OutputDataType_MP"; ZeroCross "Simulink:masks:EnableZerocrossingDetection_MP"
      mask help: Simulink:masks:CompareToConstant_MD
      mask init: same as Phase1_Mark2/Vehicle Body 3DOF External Longitudinal Wheels/Bicycle/Vehicle Body 3DOF Single Track/Signal Routing/Signal Routing/state2bus/Body Slip/div0protect - abs poly/Compare To Constant
      mask TypeOptions relop: == | ~= | < | <= | >= | >
      mask TypeOptions OutDataTypeStr: Simulink:masks:uint8 | Simulink:masks:boolean
      mask Callback ZeroCross: sl('zeroCrossEnable', gcbh);
      mask Display: disp(str)
  Fcn : Fcn  Expr=2*thresh/(3-(u(1)/thresh)^2)
  Logical Operator : Logic  AllPortsSameDT=off  OutDataTypeStr=boolean
  Switch : Switch  Criteria=u2 > Threshold  SaturateOnIntegerOverflow=off  InputSameDT=off
  y : Outport  VectorParamsAs1DForOutWhenUnconnected=off
  wires:
  Fcn/1 -> Switch/1
  Switch/1 -> y/1
  Compare To Constant1/1(y) -> Logical Operator/2
  Compare To Constant/1(y) -> Logical Operator/1
  Logical Operator/1 -> Switch/2
  u/1 -> Fcn/1, Compare To Constant/1(u), Compare To Constant1/1(u), Abs/1
  Abs/1 -> Switch/3

== system Phase1_Mark2/Vehicle Body 3DOF External Longitudinal Wheels/Bicycle/Vehicle Body 3DOF Single Track/Signal Routing/Signal Routing/state2bus/Rotation Angles to Direction Cosine Matrix/Create 3x3 Matrix ==
  M11 : Inport  PortDimensions=1
  M12 : Inport  Port=2  PortDimensions=1
  M13 : Inport  Port=3  PortDimensions=1
  M21 : Inport  Port=4  PortDimensions=1
  M22 : Inport  Port=5  PortDimensions=1
  M23 : Inport  Port=6  PortDimensions=1
  M31 : Inport  Port=7  PortDimensions=1
  M32 : Inport  Port=8  PortDimensions=1
  M33 : Inport  Port=9  PortDimensions=1
  Reshape (9) to [3x3] column-major : Reshape  OutputDimensionality=Customize  OutputDimensions=[3,3]
  Vector Concatenate : Concatenate  NumInputs=9
  Matrix : Outport  PortDimensions=[3 3]  VectorParamsAs1DForOutWhenUnconnected=off
  wires:
  M33/1 -> Vector Concatenate/9
  M23/1 -> Vector Concatenate/8
  M13/1 -> Vector Concatenate/7
  M32/1 -> Vector Concatenate/6
  Reshape (9) to [3x3] column-major/1 -> Matrix/1
  M22/1 -> Vector Concatenate/5
  M12/1 -> Vector Concatenate/4
  M31/1 -> Vector Concatenate/3
  M21/1 -> Vector Concatenate/2
  M11/1 -> Vector Concatenate/1
  Vector Concatenate/1 -> Reshape (9) to [3x3] column-major/1

== system Phase1_Mark2/Vehicle Body 3DOF External Longitudinal Wheels/Bicycle/Vehicle Body 3DOF Single Track/Signal Routing/Signal Routing/state2bus/xddot2ax/m^22gn ==
  ay : Inport  Unit=m/s^2
  ax : Inport  Port=2  Unit=m/s^2
  Unit Conversion : UnitConversion
  Unit Conversion1 : UnitConversion
  ay_g : Outport  Unit=gn  VectorParamsAs1DForOutWhenUnconnected=off
  ax_g : Outport  Port=2  Unit=gn  VectorParamsAs1DForOutWhenUnconnected=off
  wires:
  Unit Conversion1/1 -> ax_g/1
  Unit Conversion/1 -> ay_g/1
  ax/1 -> Unit Conversion1/1
  ay/1 -> Unit Conversion/1
